simulink model "PBL_model"  (R2019a)
settings: Solver=VariableStepAuto  StartTime=0.0  StopTime=10.0  RelTol=1e-3
libraries: cstblocks x1
settings Model: Creator=Nazhan  LastModifiedBy=Nazhan

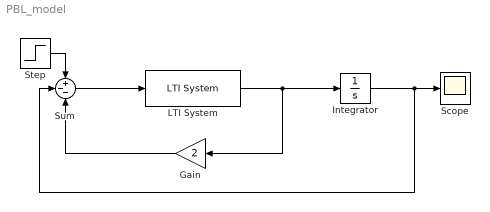
== system PBL_model ==
  Gain : Gain  Gain=2
  Integrator : Integrator
  LTI System : cstblocks/LTI System  sys=tf([20 30],[0.2 15 30 1])  IC=[]
  Scope : Scope
  Step : Step  SampleTime=0
  Sum : Sum  Inputs=+--
  wires:
  Sum/1 -> LTI System/1
  Step/1 -> Sum/1
  Gain/1 -> Sum/3
  LTI System/1 -> Gain/1, Integrator/1
  Integrator/1 -> Sum/2, Scope/1
